simulink model "CAVE_MachE_tuning"  (R2019b)
settings: configuration reference "ConfigSetDesktopFixedStep" (kept outside this file)
PreLoadFcn:
  | VSS_BICYCLE=Simulink.Variant('Dual=0');
  | VSS_DUAL=Simulink.Variant('Dual=1');
  | Dual=1;
  | load('DriveCycle2.mat')
PostLoadFcn:
  | if any(exist('dsrtsu_mdlpostloadfcn', 'file') ~= 0), dsrtsu_mdlpostloadfcn('Execute', bdroot); end
InitFcn:
  | , if any(exist('dsmpb_private', 'file') ~= 0), dsmpb_private('dsmpb_mdlclblib', 'Init', bdroot); end,
  | load('DriveCycle2.mat')
model workspace (MAT data in the model file):
  Gas = 0.383333333333
undefined symbols (not defined in the file or in its folder): AccelCmd, ActTqLF_Nm_, ActTqLR_Nm_, ActTqRF_Nm_, ActTqRR_Nm_, BattChargeLimitMaxPwr, BattChargeLimitSocBpts, BattChargeLimitTbl, BattChrgCapcty, BattDischargeLimitSocBpts, BattDischargeLimitTbl, BattDischargeMaxPwr, BattNumCellsParallel, BattNumCellsSeries, BattOpenVoltCapBpts, BattOpenVoltTbl, BattResistSocBpts, BattResistTbl, BattResistTempBpts, BrakeMaxPrs, BrakeMaxTrq, ChassisDistCg2FrontAxle, ChassisDistCg2RearAxle, ChassisVehMass, CltchCmd, CoastDown, DecelCmd, DiffRatio, DiscIntNeverNeededParam, EnvGravCnst, EnvPrs, EnvTemp, FuelSpecificGrav, GearCmd, h, InitStates, lgSw, limitedMCT, MCT, MtrEffSpdBpts, MtrEffTbl, MtrEffTrqBpts, MtrPwrMax, MtrTrqMax, pMCT, SteeringCmd, SupvsryCtrlRegenBrkCutOffTbl, SupvsryCtrlRegenSpdBpts, TestScnrioCycleNum, US06, VEH
libraries: VSIGenLib x65, simulink x46, etargetslib x38, dsmpblib x24, vehdynlibtire x12, vehdynlibsuspension x7, vehdynlibtirecommon x7, autolibshared x6, autolibutils x5, CarMaker4SL x4, VsrLibWheel x4, autolibpowerinfoutils x3
(part 13 of 13)

== stateflow chart CAVE_MachE_tuning/Vehicle Under Test/Vehicle/Actuation and Outputs/MOOG Brake Actuator/MOOG Interface/MOOG State Machine ==
  state MainStateMachine [parallel]
    settings: executionOrder=2
    state Learning
      state LearnMinStop
        en:
        state BackStopCmd
          en:
          MoogOpMode=21 ;
          PositionCmd=-100000;
        state BackStopReached
          en:
          MoogOpMode=22;
          PositionCmd=0;
        state BackStopSettle
          en:
          MoogOpMode=23;
          MinStop=ActualPosition_cnt;
          PositionCmd=0;
        (default) -> MainStateMachine.Learning.LearnMinStop.BackStopCmd
        MainStateMachine.Learning.LearnMinStop.BackStopCmd -> MainStateMachine.Learning.LearnMinStop.BackStopReached : [bitand(StatusWord,8)]
        MainStateMachine.Learning.LearnMinStop.BackStopReached -> MainStateMachine.Learning.LearnMinStop.BackStopSettle : after(2,sec)
      state StartLearning
        en:
        MoogOpMode=11;
        PositionCmd=0;
        MinStop=-200000;
        MaxStop=200000;
      state LearnMaxStop
        en:
        state BackStopCmd
          en:
          MoogOpMode=31;
          PositionCmd=100000;
        state BackStopReached
          en:
          MoogOpMode=32;
          PositionCmd=0;
        state BackStopSettle
          en:
          MoogOpMode=33;
          MaxStop=ActualPosition_cnt;
          PositionCmd=0;
        (default) -> MainStateMachine.Learning.LearnMaxStop.BackStopCmd
        MainStateMachine.Learning.LearnMaxStop.BackStopCmd -> MainStateMachine.Learning.LearnMaxStop.BackStopReached : [bitand(StatusWord,8)]
        MainStateMachine.Learning.LearnMaxStop.BackStopReached -> MainStateMachine.Learning.LearnMaxStop.BackStopSettle : after(2,sec)
      state EndLearning
        en:
        MoogOpMode=41;
        PositionCmd=0;
        LearningComplete=1;
        FaultCntr=0;
      (default) -> StartLearning
      StartLearning -> LearnMinStop : after(0.5,sec)[InitComplete ==1]
      LearnMinStop -> LearnMaxStop : after(1,sec)[InitComplete ==1  && MinStop ~=-200000]
      LearnMaxStop -> EndLearning : after(1,sec)[InitComplete ==1  && MaxStop ~=200000 && ((MaxStop-MinStop)>ActuatorMinTravelForReady)]
    state NormalOperation
      state LearningNotComplete
        en:
        MoogOpMode=101;
        Actuator_Ready=0;
        du:
        PositionCmd=0;
      state LearningComplete
        en:
        MoogOpMode=102;
        Actuator_Ready=1;
        du:
        PositionCmd=TargetPosition_cnt;
      (default) -> LearningNotComplete
      LearningNotComplete -> LearningComplete : after(1,sec)[LearningComplete==1]
    MainStateMachine.Learning.LearnMaxStop.BackStopSettle -> NormalOperation : after(10,sec)
    Learning -> NormalOperation : after(1,sec)[LearningComplete==1]
    NormalOperation -> Learning : [PositionLearningTrigger==1]{Actuator_Ready =0;
        | LearningComplete=0}
    (default) -> NormalOperation : {Actuator_Ready =0;
        | LearningComplete=0}
  state MoogStateMachine [parallel]
    settings: executionOrder=1
    state Initialisation
      state SwitchOffDisabled
        % StatusWord= xxxx_xxxx_x0xx_0000, 0x00, 0d
        en:
        MoogSMState=13;
        ControlWord=0; % 0x00
      state Init
        en:
        MoogSMState=11;
        ControlWord=0;
        InitComplete =0;
      state ClearFault
        en:
        MoogSMState=12;
        ControlWord=128; % 0x80
      state SwitchOnDisabled
        % StatusWord= xxxx_xxxx_x1xx_0000, 0x40, 64d
        en:
        MoogSMState=14;
        ControlWord=6; % 0x06
      state ReadyToSwitchOn
        % StatusWord=xxxx_xxxx_x01x_0001, 0x21, 33d
        en:
        MoogSMState=15;
        ControlWord=7; % 0x07
      state SwitchedOn
        % StatusWord=xxxx_xxxx_x01x_0011, 0x23, 35d
        en:
        MoogSMState=16;
        ControlWord=15; % 0x0F
      state OperationEnabled
        % StatusWord=xxxx_xxxx_x01x_0111, 0x27, 39d
        en:
        MoogSMState=17;
        ControlWord=15; % 0x0F
        InitComplete=1;
      SwitchOffDisabled -> Init [order 2] : after(1,sec)[bitand(StatusWord,8)]{FaultCntr=FaultCntr+1;}
      (default) -> Init
      Init -> ClearFault : after(0.5,sec)
      ClearFault -> SwitchOffDisabled : after(0.5,sec)
      SwitchOffDisabled -> SwitchOnDisabled [order 1] : after(0.1,sec)[bitand(StatusWord,64)]
      OperationEnabled -> Init : after(1,sec)[bitand(StatusWord,8)]{FaultCntr=FaultCntr+1;}
      SwitchedOn -> Init [order 2] : after(1,sec)[bitand(StatusWord,8)]{FaultCntr=FaultCntr+1;}
      ReadyToSwitchOn -> Init [order 2] : after(1,sec)[bitand(StatusWord,8)]{FaultCntr=FaultCntr+1;}
      SwitchOnDisabled -> Init [order 2] : after(1,sec)[bitand(StatusWord,8)]{FaultCntr=FaultCntr+1;}
      SwitchOnDisabled -> ReadyToSwitchOn [order 1] : after(0.1,sec)[bitand(StatusWord,32) &...
          |  bitand(StatusWord,1)]
      ReadyToSwitchOn -> SwitchedOn [order 1] : after(0.1,sec)[bitand(StatusWord,32) & ...
          | bitand(StatusWord,2) & ...
          | bitand(StatusWord,1)]
      SwitchedOn -> OperationEnabled [order 1] : after(0.1,sec)[bitand(StatusWord,32) & ...
          | bitand(StatusWord,4) & ...
          | bitand(StatusWord,2) & ...
          | bitand(StatusWord,1)]
    state Wait
      en:
      MoogSMState=31;
      Actuator_Ready=0;
      InitComplete =0;
      LearningComplete=0;
    state PositionControl
      state EnableSetPoint
        en:
        MoogSMState=21;
        ControlWord=47; % 0x2F
      state BeginMotion
        en:
        MoogSMState=22;
        ControlWord=63; % 0x3F
      (default) -> EnableSetPoint
      EnableSetPoint -> BeginMotion : after(0.001,sec)[Actuator_Ready==1 || ...
          | MoogOpMode==21 || ...
          | MoogOpMode==31]
      BeginMotion -> EnableSetPoint : after(0.001,sec)
    Initialisation -> Wait [order 2] : after(2,sec)[CAN_CommsOK_Flg ==0]
    (default) -> Initialisation : {FaultCntr=0;}
    Initialisation -> Wait [order 3] : [FaultCntr>=5]
    Wait -> Initialisation : [ResetCmd &&CAN_CommsOK_Flg==1 ]{Actuator_Ready=0;FaultCntr=0;}
    Initialisation -> PositionControl [order 1] : [InitComplete==1]
    PositionControl -> Initialisation [order 1] : [ResetCmd ]{InitComplete=0;}
    PositionControl -> Initialisation [order 2] : [bitand(StatusWord,8)]{InitComplete=0;FaultCntr=FaultCntr+1;}
  data: CAN_CommsOK_Flg input; ControlWord output; PositionCmd output; ResetCmd input; PositionLearningTrigger input; StatusWord input; Actuator_Ready output; FaultCntr output; MoogSMState output; InitComplete output; MoogOpMode output; LearningComplete output; ActualPosition_cnt input; MaxStop output; MinStop output; TargetPosition_cnt input; ActuatorMinTravelForReady input

== matlab function CAVE_MachE_tuning/Vehicle Under Test/Vehicle/Rototest and ORNL Interface/Get Wheel Spd Cmd Based on Wheel Dynamics/Whl Dynamics & Format CM Powertrain Signal/Subsystem/MATLAB Function ==
  data: axleTorq input; switchFlag output; wheelSpd input
function switchFlag = fcn(axleTorq, wheelSpd)

% if braking and vehicle has stopped
if (abs(axleTorq) < 1e-5 && abs(wheelSpd) < 1e-5)
    switchFlag = 1;
else
    switchFlag = 0;
end

== matlab function CAVE_MachE_tuning/Vehicle Under Test/Vehicle/Rototest and ORNL Interface/Get Wheel Spd Cmd Based on Wheel Dynamics/Whl Dynamics & Format CM Powertrain Signal/Subsystem2/MATLAB Function ==
  data: axleTorq input; switchFlag output; wheelSpd input
function switchFlag = fcn(axleTorq, wheelSpd)

% if braking and vehicle has stopped
if (abs(axleTorq) < 1e-5 && abs(wheelSpd) < 1e-5)
    switchFlag = 1;
else
    switchFlag = 0;
end

== matlab function CAVE_MachE_tuning/Vehicle Under Test/Vehicle/Rototest and ORNL Interface/Get Wheel Spd Cmd Based on Wheel Dynamics/Whl Dynamics & Format CM Powertrain Signal/Subsystem3/MATLAB Function ==
  data: axleTorq input; switchFlag output; wheelSpd input
function switchFlag = fcn(axleTorq, wheelSpd)

% if braking and vehicle has stopped
if (abs(axleTorq) < 1e-5 && abs(wheelSpd) < 1e-5)
    switchFlag = 1;
else
    switchFlag = 0;
end

== matlab function CAVE_MachE_tuning/Vehicle Under Test/Vehicle/Vehicle Dynamics/Vehicle 14DOF/Wheels and Tires/VDBS/Tires/MF Tires/MATLAB Function ==
  data: axleTorq input; switchFlag output; wheelSpd input
function switchFlag = fcn(axleTorq, wheelSpd)

% if braking and vehicle has stopped
%if (abs(axleTorq) < 1e-5 && abs(wheelSpd) < 1e-5)
if abs(wheelSpd) < 1e-5
    switchFlag = 1;
else
    switchFlag = 0;
end

== matlab function CAVE_MachE_tuning/Vehicle Under Test/Vehicle/Vehicle Dynamics/Vehicle 14DOF/Wheels and Tires/VDBS/Tires/MF Tires/MATLAB Function1 ==
  data: axleTorq input; switchFlag output; wheelSpd input
function switchFlag = fcn(axleTorq, wheelSpd)

% if braking and vehicle has stopped
%if (abs(axleTorq) < 1e-5 && abs(wheelSpd) < 1e-5)
if abs(wheelSpd) < 1e-5
    switchFlag = 1;
else
    switchFlag = 0;
end

== matlab function CAVE_MachE_tuning/Vehicle Under Test/Vehicle/Rototest and ORNL Interface/Get Wheel Spd Cmd Based on Wheel Dynamics/Whl Dynamics & Format CM Powertrain Signal/Subsystem4/MATLAB Function ==
  data: axleTorq input; switchFlag output; wheelSpd input
function switchFlag = fcn(axleTorq, wheelSpd)

% if braking and vehicle has stopped
if (abs(axleTorq) < 1e-5 && abs(wheelSpd) < 1e-5)
    switchFlag = 1;
else
    switchFlag = 0;
end

== stateflow chart CAVE_MachE_tuning/Vehicle Under Test/Vehicle/Rototest and ORNL Interface/To Rototest with Band-Aid/Band-Aid/Band-Aid ==
  state dStop
    en:
    OutMode = 0;
    State = 3;
  state Running
    state SpeedMode
      en:
      OutMode = 1;
      state Blend
        en:
        OutSpd = InSpd;
        State = 0.1;
      state Driving
        du:
        OutSpd = InSpd;
        State = 0.2;
      (default) -> Blend
      Blend -> Driving
    state TorqueMode
      en:
      OutMode = 0;
      du:
      State = 1;
    (default) -> SpeedMode
    TorqueMode -> Blend : [after(SettleTime, sec) || ...
        | ~BrkSw]
    SpeedMode -> TorqueMode : [(any(InSpd < SpdLatchThr) && ...
        | (VehSpd_kph < VehSpdThr_kph) && BrkSw)]
  note: The vehicle will enter speed mode (driving) if:
      | The vehicle has been in torque mode for a calibrated time (settleTime) AND
      | The Input Speed (InSpd) is greater than a Launch Treshold (LaunchSpdThr) OR
      | The Input Torque (InTrq) is greater than calibrated torque value (LaunchTrqThr).
      | Criteria 1) sees the dyno has "settled" and allows the dyno to go back into speed mode.
      | Criteria 2) sees the vehicle is attempting to reaccelerate and pushes into speed mode.
      |
      | The vehicle will enter torque mode (zero) if:
      | Input Speed (InSpd) goes below the calibrated speed (SpdLatchThr) AND
      | Brake (BrkSw) is active.
      | 2) dStop is activated.
      | Criteria 1) sees the vehicle is attempting to come to a stop and unloads the dyno.
      | Criteria 2) is SHTF.
      |
      | && ...
      | (InSpd > LaunchSpdThr || ...
      | InTrq > LaunchTrqThr)
  (default) -> dStop
  Running -> dStop : [dStop]
  dStop -> Running : [~dStop]
  data: LaunchSpdThr input; LaunchTrqThr input; SpdLatchThr input; BrkSw input; InSpd input; InTrq input; OutMode output size=1; OutSpd output; State output; SettleTime input; dStop input; VehSpd_kph input; VehSpdThr_kph input

== matlab function CAVE_MachE_tuning/Vehicle Under Test/Vehicle/Rototest and ORNL Interface/To Rototest with Band-Aid/RotoTestEthTx/MATLAB Function ==
  data: SpTqRR input; y output; SpTqLR input; SpTqRF input; SpTqLF input; SystemActive input
function y = fcn(SpTqRR, SpTqLR, SpTqRF, SpTqLF, SystemActive)

y = 0;
if SpTqRR == 1 && SystemActive == 0
    y = 30;
elseif SpTqRR == 0 && SystemActive == 0
    y = 0;
elseif SpTqRR == 1 && SystemActive == 1
    y = 31;
elseif SpTqRR == 0 && SystemActive == 1
    y = 1;
end

y = uint8(y);

== matlab function CAVE_MachE_tuning/Vehicle Under Test/Vehicle/Vehicle Dynamics/Vehicle 14DOF/Wheels and Tires/VDBS/Tires/MF Tires/MATLAB Function2 ==
  data: axleTorq input; switchFlag output; wheelSpd input
function switchFlag = fcn(axleTorq, wheelSpd)

% if braking and vehicle has stopped
%if (abs(axleTorq) < 1e-5 && abs(wheelSpd) < 1e-5)
if abs(wheelSpd) < 1e-5
    switchFlag = 1;
else
    switchFlag = 0;
end

== matlab function CAVE_MachE_tuning/Vehicle Under Test/Vehicle/Vehicle Dynamics/Vehicle 14DOF/Wheels and Tires/VDBS/Tires/MF Tires/MATLAB Function3 ==
  data: axleTorq input; switchFlag output; wheelSpd input
function switchFlag = fcn(axleTorq, wheelSpd)

% if braking and vehicle has stopped
%if (abs(axleTorq) < 1e-5 && abs(wheelSpd) < 1e-5)
if abs(wheelSpd) < 1e-5
    switchFlag = 1;
else
    switchFlag = 0;
end
